simulink library "dpd_lib"  (Simulink 8.7)
settings: Solver=ode45  StartTime=0.0  StopTime=10.0  RelTol=1e-3
PreLoadFcn:
  | LutContent = LUTS.ENTRIES;
InitFcn:
  | LutContent = LUTS.ENTRIES;
undefined symbols (not defined in the file): AdvDSPBChannelOutDisplay, AdvDSPBDMemDisplay, cordic_gain, dpoly, dspba_ChannelInVis, dspba_ChannelOutVis, dspba_internal_get_channel_ports, evalAionMaskParam, latency, LUTS, primtype, UseDontCare, value
libraries: DSPBAPrim x49, dpd_lib x33, DSPBAVectorUtil x2, DSPBABase x1, CORDIC_lib x1
settings Model: Creator=VMAUER  LastModifiedBy=5g

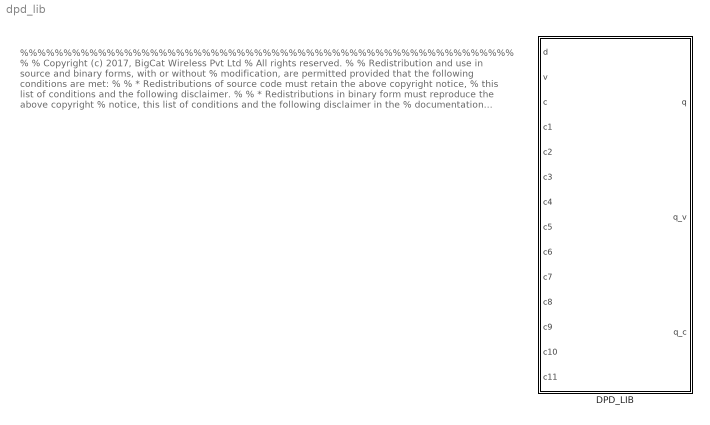
== system dpd_lib ==
  note: %%%%%%%%%%%%%%%%%%%%%%%%%%%%%%%%%%%%%%%%%%%%%%%%%%%%%%%%%
      |  %
      |  % Copyright (c) 2017, BigCat Wireless Pvt Ltd
      |  % All rights reserved.
      |  %
      |  % Redistribution and use in source and binary forms, with or without
      |  % modification, are permitted provided that the following conditions are met:
      |  %
      |  %     * Redistributions of source code must retain the above copyright notice,
      |  %       this list of conditions and the following disclaimer.
      |  %
      |  %     * Redistributions in binary form must reproduce the above copyright
      |  %       notice, this list of conditions and the following disclaimer in the
      |  %       documentation and/or other materials provided with the distribution.
      |  %
      |  %     * Neither the name of the copyright holder nor the names of its contributors
      |  %       may be used to endorse or promote products derived from this software
      |  %       without specific prior written permission.
      |  %
      |  %
      |  %
      |  % THIS SOFTWARE IS PROVIDED BY THE COPYRIGHT HOLDERS AND CONTRIBUTORS "AS IS"
      |  % AND ANY EXPRESS OR IMPLIED WARRANTIES, INCLUDING, BUT NOT LIMITED TO, THE
      |  % IMPLIED WARRANTIES OF MERCHANTABILITY AND FITNESS FOR A PARTICULAR PURPOSE ARE
      |  % DISCLAIMED. IN NO EVENT SHALL THE COPYRIGHT HOLDER OR CONTRIBUTORS BE LIABLE
      |  % FOR ANY DIRECT, INDIRECT, INCIDENTAL, SPECIAL, EXEMPLARY, OR CONSEQUENTIAL
      |  % DAMAGES (INCLUDING, BUT NOT LIMITED TO, PROCUREMENT OF SUBSTITUTE GOODS OR
      |  % SERVICES; LOSS OF USE, DATA, OR PROFITS; OR BUSINESS INTERRUPTION) HOWEVER
      |  % CAUSED AND ON ANY THEORY OF LIABILITY, WHETHER IN CONTRACT, STRICT LIABILITY,
      |  % OR TORT (INCLUDING NEGLIGENCE OR OTHERWISE) ARISING IN ANY WAY OUT OF THE USE
      |  % OF THIS SOFTWARE, EVEN IF ADVISED OF THE POSSIBILITY OF SUCH DAMAGE.
      |  %
      |   %%%%%%%%%%%%%%%%%%%%%%%%%%%%%%%%%%%%%%%%%%%%%%%%%%%%%%%%%%
  DPD_LIB : Subsystem  mask{CoefWidth=16, Coeff_fractionwidth=11, DataWidth=16, fractionwidth=15, Lateny=0, ClockMargin=0, Pipeline_stages=0, LutContent=0}
      mask prompts: CoefWidth "Coefficient Width"; DataWidth "Data Width"; LutContent "initial Lut Content"
      mask Display:
      | disp('DPD');
      | port_label('input',1,'d');
      | port_label('input',2,'v');
      | port_label('input',3,'c');
      | port_label('input',4,'coeffs1');
      | port_label('input',5,'coeffs2');
      | port_label('input',6,'coeffs3');
      | port_label('input',7,'coeffs4');
      | port_label('input',8,'coeffs5');
      | port_label('input',9,'coeffs6');
      | port_label('input',10,'coeffs7');
      | port_label('input',11,'coeffs8');
      | port_label('input',12,'LUTAddress');
      | port_label('input',13,'RegField1');
      | port_label('input',14,'Predistorter_Enable');
      | port_label('output',1,'q');
      | port_label('output',2,'q_v');
      | port_label('output',3,'q_c');

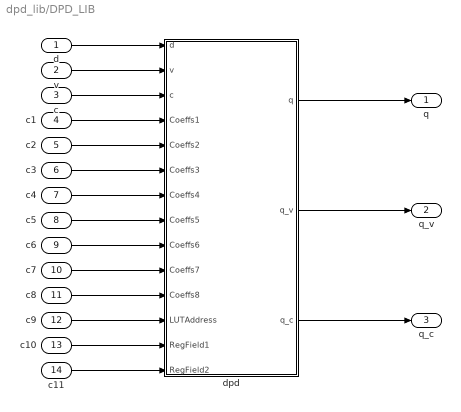
== system dpd_lib/DPD_LIB ==
  d : Inport
  v : Inport  Port=2
  c : Inport  Port=3
  c1 : Inport  Port=4
  c2 : Inport  Port=5
  c3 : Inport  Port=6
  c4 : Inport  Port=7
  c5 : Inport  Port=8
  c6 : Inport  Port=9
  c7 : Inport  Port=10
  c8 : Inport  Port=11
  c9 : Inport  Port=12
  c10 : Inport  Port=13
  c11 : Inport  Port=14
  dpd : Subsystem
  q : Outport
  q_v : Outport  Port=2
  q_c : Outport  Port=3
  wires:
  c/1 -> dpd/3(c)
  d/1 -> dpd/1(d)
  v/1 -> dpd/2(v)
  dpd/1(q) -> q/1
  dpd/2(q_v) -> q_v/1
  dpd/3(q_c) -> q_c/1
  c1/1 -> dpd/4(Coeffs1)
  c2/1 -> dpd/5(Coeffs2)
  c3/1 -> dpd/6(Coeffs3)
  c4/1 -> dpd/7(Coeffs4)
  c5/1 -> dpd/8(Coeffs5)
  c6/1 -> dpd/9(Coeffs6)
  c7/1 -> dpd/10(Coeffs7)
  c10/1 -> dpd/13(RegField1)
  c9/1 -> dpd/12(LUTAddress)
  c8/1 -> dpd/11(Coeffs8)
  c11/1 -> dpd/14(RegField2)

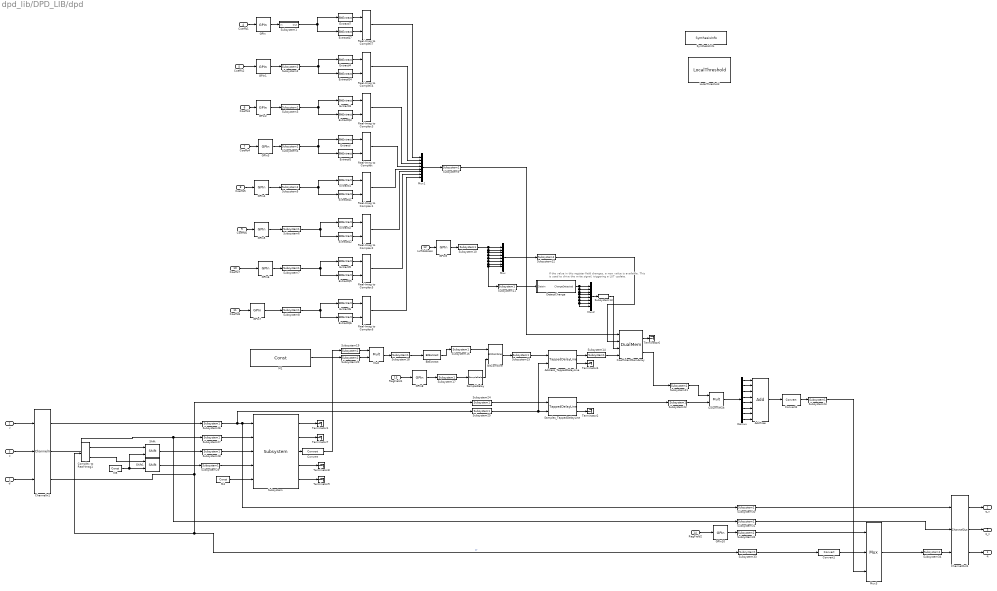
== system dpd_lib/DPD_LIB/dpd ==
  note: If the value in this register field changes, a new value is available.
      | This is used to drive the write signal, triggering a LUT update.
  d : Inport
  v : Inport  Port=2
  c : Inport  Port=3
  Coeffs1 : Inport  Port=4
  Coeffs2 : Inport  Port=5
  Coeffs3 : Inport  Port=6
  Coeffs4 : Inport  Port=7
  Coeffs5 : Inport  Port=8
  Coeffs6 : Inport  Port=9
  Coeffs7 : Inport  Port=10
  Coeffs8 : Inport  Port=11
  LUTAddress : Inport  Port=12
  RegField1 : Inport  Port=13
  RegField2 : Inport  Port=14
  AddTree : DSPBAPrim/Add  primtype=add  nInputs=evalAionMaskParam(gcb,'value',1)  nOutputs=1  omode=Inherit via internal rule with word growth  otype=sfix(16)  scale=2^-15  rndmethod=Unbiased  factor=1  satmethod=Symmetric  shift_vec=[0 1 2 -1]  value=8  inPortNames=[' '; ' ';]  outPortNames=[' ']  dspbaimage=dspba_prim.jpg  text=fprintf('+');  style=Optimised  visibilities=1032+2^17+2^18+2^19  genFPC=off  floatRounding=correct  advOptions=[]  version=20130821
  Address_TappedDelayLine : DSPBAVectorUtil/TappedDelayLine  numTaps=size(LutContent, 2)  zeroOrOne=0  reverse=off
  BitCombine : DSPBAPrim/BitCombine  primtype=bitcombine  nInputs=2  nOutputs=1  omode=Inherit via internal rule  otype=sfix(16)  scale=2^-15  rndmethod=Unbiased  factor=1  satmethod=Symmetric  shift_vec=[0 1 2 -1]  value=0  inPortNames=['l'; 'h';]  outPortNames=[' ']  dspbaimage=dspba_prim.jpg  text=fprintf('[h,l]');  style=Optimised  visibilities=8+2  version=20090407
  BitExtract : DSPBAPrim/BitExtract  primtype=bitextract  nInputs=1  nOutputs=1  omode=Specify via dialog  otype=ufix(8)  scale=1  rndmethod=Unbiased  factor=1  satmethod=Symmetric  shift_vec=[0 1 2 -1]  value=log2(size(LutContent,1))  inPortNames=[' '; ' ';]  outPortNames=[' ']  dspbaimage=dspba_prim.jpg  text=fprintf('..%d', value);  style=Optimised  visibilities=8 + 1024  version=20090407
  ChannelIn1 : DSPBAPrim/ChannelIn  primtype=channelin  nInputs=dspba_internal_get_channel_ports(gcb)  nOutputs=dspba_internal_get_channel_ports(gcb)  omode=Inherit via internal rule  otype=sfix(16)  scale=2^-15  rndmethod=Unbiased  factor=1  satmethod=Symmetric  shift_vec=[0 1 2 -1]  value=1  inPortNames=['v'; 'c'; '0'; '1'; '2'; '3'; '4'; '5'; '6'; '7'; '8'; '9'; 'A'; 'B'; 'D'; 'E'; 'F'; 'G'; 'H'; 'I'; 'J'; 'K'; 'L'; 'M'; 'N'; 'O'; 'P'; 'Q'; 'R'; 'S'; 'T'; 'U'; 'W'; 'X'; 'Y'; 'Z']  outPortNames=['v'; 'c'; '0'; '1'; '2'; '3'; '4'; '5'; '6'; '7'; '8'; '9'; 'A'; 'B'; 'D'; 'E'; 'F'; 'G'; 'H'; 'I'; 'J'; 'K'; 'L'; 'M'; 'N'; 'O'; 'P'; 'Q'; 'R'; 'S'; 'T'; 'U'; 'W'; 'X'; 'Y'; 'Z']  dspbaimage=dspba_prim.jpg  text=fprintf('In');  style=Optimised  dataSignals=1  foldingEnabled=off  channels=1  sampleRate=200  packetBeginPresent=off  packetBeginEnabled=off  visibilities=dspba_ChannelInVis(gcb)  latencyCorrection=0  version=20141013
  ChannelOut1 : DSPBAPrim/ChannelOut  primtype=channelout  nInputs=dspba_internal_get_channel_ports(gcb)  nOutputs=dspba_internal_get_channel_ports(gcb)  omode=Inherit via internal rule  otype=sfix(16)  scale=2^-15  rndmethod=Unbiased  factor=1  satmethod=Symmetric  shift_vec=[0 1 2 -1]  value=1  inPortNames=['v'; 'c'; '0'; '1'; '2'; '3'; '4'; '5'; '6'; '7'; '8'; '9'; 'A'; 'B'; 'D'; 'E'; 'F'; 'G'; 'H'; 'I'; 'J'; 'K'; 'L'; 'M'; 'N'; 'O'; 'P'; 'Q'; 'R'; 'S'; 'T'; 'U'; 'W'; 'X'; 'Y'; 'Z']  outPortNames=['v'; 'c'; '0'; '1'; '2'; '3'; '4'; '5'; '6'; '7'; '8'; '9'; 'A'; 'B'; 'D'; 'E'; 'F'; 'G'; 'H'; 'I'; 'J'; 'K'; 'L'; 'M'; 'N'; 'O'; 'P'; 'Q'; 'R'; 'S'; 'T'; 'U'; 'W'; 'X'; 'Y'; 'Z']  dspbaimage=dspba_prim.jpg  text=fprintf('Out%s', AdvDSPBChannelOutDisplay(latency));  style=Optimised  dataSignals=1  foldingEnabled=off  channels=1  sampleRate=200  packetBeginPresent=off  packetBeginEnabled=off  visibilities=dspba_ChannelOutVis(gcb)  latency=101  latencyCorrection=0  version=20141013
  CoefficientMemArray : DSPBAPrim/DualMem  primtype=dualmem  nInputs=4  nOutputs=2  omode=Specify via dialog  otype=sfix(CoefWidth)  scale=2^-Coeff_fractionwidth  rndmethod=Unbiased  factor=1  satmethod=Symmetric  shift_vec=[0 1 2 -1]  value=[LUTS.ENTRIES' LUTS.ENTRIES']'  inPortNames=['d1'; 'a1'; 'w1'; 'a2']  outPortNames=['q1'; 'q2']  dspbaimage=dspba_prim.jpg  text=fprintf('dmem%s',AdvDSPBDMemDisplay(UseDontCare));  style=Optimised  visibilities=8 + 1024 + 2^17  UseDontCare=on  TwinWritePorts=off  version=20141001
  ColumnMult : DSPBAPrim/Mult  primtype=mult  nInputs=2  nOutputs=1  omode=Inherit via internal rule  otype=sfix(16)  scale=2^-11  rndmethod=Unbiased  factor=1  satmethod=Symmetric  shift_vec=[0 1 2 -1]  value=0  inPortNames=[' '; ' ';]  outPortNames=[' ']  dspbaimage=dspba_prim.jpg  text=fprintf('X');  style=Optimised  visibilities=8+2^18+2^19  floatPrecision=float32_m23  floatRounding=correct  advOptions=[]  version=20130115
  Complex to Real-Imag1 : ComplexToRealImag
  Convert : DSPBAPrim/Convert  primtype=convert  nInputs=1  nOutputs=1  omode=Specify via dialog  otype=ufix(10)  scale=2^-8  rndmethod=Truncate  factor=1  satmethod=None  shift_vec=[0 1 2 -1]  value=round([0:255]/17)  inPortNames=[' '; ' ';]  outPortNames=[' '; 'c']  dspbaimage=dspba_prim.jpg  text=fprintf('convert');  style=Optimised  visibilities=8+64+256+2^17  clipdetect=off  floatPrecision=float32_m23  advOptions=[]  version=20130211
  Convert1 : DSPBAPrim/Convert  primtype=convert  nInputs=1  nOutputs=1  omode=Specify via dialog  otype=sfix(16)  scale=2^-15  rndmethod=Unbiased  factor=1  satmethod=None  shift_vec=[0 1 2 -1]  value=round([0:255]/17)  inPortNames=[' '; ' ';]  outPortNames=[' '; 'c']  dspbaimage=dspba_prim.jpg  text=fprintf('convert');  style=Optimised  visibilities=8+64+256+2^17  clipdetect=off  floatPrecision=float32_m23  advOptions=[]  version=20130211
  Convert2 : DSPBAPrim/Convert  primtype=convert  nInputs=1  nOutputs=1  omode=Specify via dialog  otype=sfix(DataWidth)  scale=2^-fractionwidth  rndmethod=Unbiased  factor=1  satmethod=None  shift_vec=[0 1 2 -1]  value=round([0:255]/17)  inPortNames=[' '; ' ';]  outPortNames=[' '; 'c']  dspbaimage=dspba_prim.jpg  text=fprintf('convert');  style=Optimised  visibilities=8+64+256  clipdetect=off  floatPrecision=float32_m23  advOptions=[]  version=20130211
  Demux : Demux  Outputs=8
  DetectChange : Subsystem
  ExtractI{,1..7} (8 alike) : DSPBAPrim/BitExtract  primtype=bitextract  nInputs=1  nOutputs=1  omode=Specify via dialog  otype=sfix(CoefWidth)  scale=2^-Coeff_fractionwidth  rndmethod=Unbiased  factor=1  satmethod=Symmetric  shift_vec=[0 1 2 -1]  value=CoefWidth  inPortNames=[' '; ' ';]  outPortNames=[' ']  dspbaimage=dspba_prim.jpg  text=fprintf('..%d', value);  style=Optimised  visibilities=8 + 1024  version=20090407
  ExtractQ{,1..3,5..6} (6 alike) : DSPBAPrim/BitExtract  primtype=bitextract  nInputs=1  nOutputs=1  omode=Specify via dialog  otype=sfix(CoefWidth)  scale=2^-Coeff_fractionwidth  rndmethod=Unbiased  factor=1  satmethod=Symmetric  shift_vec=[0 1 2 -1]  value=0  inPortNames=[' '; ' ';]  outPortNames=[' ']  dspbaimage=dspba_prim.jpg  text=fprintf('..%d', value);  style=Optimised  visibilities=8 + 1024  version=20090407
  ExtractQ4 : DSPBAPrim/BitExtract  primtype=bitextract  nInputs=1  nOutputs=1  omode=Specify via dialog  otype=sfix(DataWidth)  scale=2^-Coeff_fractionwidth  rndmethod=Unbiased  factor=1  satmethod=Symmetric  shift_vec=[0 1 2 -1]  value=0  inPortNames=[' '; ' ';]  outPortNames=[' ']  dspbaimage=dspba_prim.jpg  text=fprintf('..%d', value);  style=Optimised  visibilities=8 + 1024  version=20090407
  ExtractQ7 : DSPBAPrim/BitExtract  primtype=bitextract  nInputs=1  nOutputs=1  omode=Specify via dialog  otype=sfix(DataWidth)  scale=2^-Coeff_fractionwidth  rndmethod=Unbiased  factor=1  satmethod=Symmetric  shift_vec=[0 1 2 -1]  value=0  inPortNames=[' '; ' ';]  outPortNames=[' ']  dspbaimage=dspba_prim.jpg  text=fprintf('..%d', value);  style=Optimised  visibilities=8 + 1024  version=20090407
  GPIn{,1..10} (11 alike) : DSPBAPrim/GPIn  primtype=gpin  nInputs=evalAionMaskParam(gcb,'value',1)  nOutputs=evalAionMaskParam(gcb,'value',1)  omode=Inherit via internal rule  otype=sfix(16)  scale=2^-15  rndmethod=Unbiased  factor=1  satmethod=Symmetric  shift_vec=[0 1 2 -1]  value=1  inPortNames=[' ' ' ' ' ' ' ' ' ' ' ' ' ' ' ' ' ' ' ' ' ' ' ' ' ' ' ' ' ' ' ' ' ' ' ' ' ' ' ' ' ' ' ' ' ' ' ' ' ' ' ' ' ' ' ' ' ' ' ' ' ' ' ' ' ' ' ' ' ']'  outPortNames=[' ' ' ' ' ' ' ' ' ' ' ' ' ' ' ' ' ' ' ' ' ' ' ' ' ' ' ' ' ' ' ' ' ' ' ' ' ' ' ' ' ' ' ' ' ' ' ' ' ' ' ' ' ' ' ' ' ' ' ' ' ' ' ' ' ' ' ' ' ']'  dspbaimage=dspba_prim.jpg  text=fprintf('GPIn');  style=Optimised  visibilities=1024  latencyCorrection=0  version=20090407
  LocalThreshold : DSPBABase/LocalThreshold  margin=ClockMargin  delayRegOrRAMThresholdBits=-1  MediumDualMemThresholdBits=-1  LargeDualMemThresholdBits=-1  hardMultiplierThresholdLuts=-1  complexMultKaratsuba=off  version=0
  M1 : DSPBAPrim/Const  primtype=const  nInputs=0  nOutputs=1  omode=Specify via dialog  otype=uint(8)  scale=1  rndmethod=Unbiased  factor=1  satmethod=Symmetric  shift_vec=[0 1 2 -1]  value=size(LutContent, 1) * (1/cordic_gain)  inPortNames=['+'; '+';]  outPortNames=[' ']  dspbaimage=dspba_prim.jpg  text=fprintf('%s', num2str(value));  style=Optimised  visibilities=8 + 1024  floatPrecision=float32_m23  version=20120820
  M4 : DSPBAPrim/Const  primtype=const  nInputs=0  nOutputs=1  omode=Specify via dialog  otype=sfix(16)  scale=2^-15  rndmethod=Unbiased  factor=1  satmethod=Symmetric  shift_vec=[0 1 2 -1]  value=0  inPortNames=['+'; '+';]  outPortNames=[' ']  dspbaimage=dspba_prim.jpg  text=fprintf('%s', num2str(value));  style=Optimised  visibilities=8 + 1024  floatPrecision=float32_m23  version=20120820
  M5 : DSPBAPrim/Const  primtype=const  nInputs=0  nOutputs=1  omode=Specify via dialog  otype=uint(4)  scale=2^0  rndmethod=Unbiased  factor=1  satmethod=Symmetric  shift_vec=[0 1 2 -1]  value=2  inPortNames=['+'; '+';]  outPortNames=[' ']  dspbaimage=dspba_prim.jpg  text=fprintf('%s', num2str(value));  style=Optimised  visibilities=8 + 1024  floatPrecision=float32_m23  version=20120820
  Mult : DSPBAPrim/Mult  primtype=mult  nInputs=2  nOutputs=1  omode=Inherit via internal rule  otype=double  scale=1  rndmethod=Unbiased  factor=1  satmethod=Symmetric  shift_vec=[0 1 2 -1]  value=0  inPortNames=[' '; ' ';]  outPortNames=[' ']  dspbaimage=dspba_prim.jpg  text=fprintf('X');  style=Optimised  visibilities=8  floatPrecision=float32_m23  floatRounding=correct  advOptions=[]  version=20130115
  Mux : Mux  Inputs=8
  Mux1 : Mux  Inputs=8
  Mux2 : Mux  Inputs=8
  Mux3 : DSPBAPrim/Mux  primtype=mux  nInputs=evalAionMaskParam(gcb,'value',1)+1  nOutputs=1  omode=Inherit via internal rule  otype=sfix(16)  scale=2^-15  rndmethod=Unbiased  factor=1  satmethod=Symmetric  shift_vec=[0 1 2 -1]  value=2  inPortNames=['s'; 'd0'; 'd1'; 'd2'; 'd3'; 'd4'; 'd5'; 'd6'; 'd7'; 'd8'; 'd9';]  outPortNames=[' ']  dspbaimage=dspba_prim.jpg  text=fprintf('%s', primtype);  style=Optimised  visibilities=1032  version=20131025
  Real-Imag to Complex{,1..7} (8 alike) : RealImagToComplex
  SampleDelay : DSPBAPrim/SampleDelay  primtype=sampdelay  nInputs=1  nOutputs=1  omode=Inherit via internal rule  otype=sfix(16)  scale=2^-15  rndmethod=Unbiased  factor=1  satmethod=Symmetric  shift_vec=[0 1 2 -1]  value=1  inPortNames=[' '; ' ';]  outPortNames=[' ']  dspbaimage=dspba_prim.jpg  text=dpoly(1, eye(1,value+1), 'z')  style=Optimised  visibilities=8 + 1024 + 2^17 + 2^18  flexible=off  slackgroup=0  augmented=0  version=20090407  advOptions=[]
  Samples_TappedDelayLine : DSPBAVectorUtil/TappedDelayLine  numTaps=size(LutContent, 2)  zeroOrOne=0  reverse=off
  Shift : DSPBAPrim/Shift  primtype=shift  nInputs=2  nOutputs=1  omode=Specify via dialog  otype=sfix(16)  scale=2^-15  rndmethod=Unbiased  factor=1  satmethod=Symmetric  shift_vec=[0 1 2 -1]  value=0  inPortNames=['a'; 'b';]  outPortNames=[' ']  dspbaimage=dspba_prim.jpg  text=fprintf('a >> b');  style=Optimised  visibilities=8  version=20090407
  Shift1 : DSPBAPrim/Shift  primtype=shift  nInputs=2  nOutputs=1  omode=Specify via dialog  otype=sfix(16)  scale=2^-15  rndmethod=Unbiased  factor=1  satmethod=Symmetric  shift_vec=[0 1 2 -1]  value=0  inPortNames=['a'; 'b';]  outPortNames=[' ']  dspbaimage=dspba_prim.jpg  text=fprintf('a >> b');  style=Optimised  visibilities=8  version=20090407
  Subsystem : CORDIC_lib/Subsystem  stages=stages  angle_bits=xy_angle_bits  angle_frac_bits=xy_angle_fract_bits  xy_bits=xy_bits  xy_frac_bits=xy_fract_bits
  Subsystem1 : Subsystem
  Subsystem{2..34} (33 alike) : dpd_lib/DPD_LIB/dpd/Subsystem1
  SynthesisInfo : DSPBAPrim/SynthesisInfo  primtype=synthinfo  nInputs=0  nOutputs=0  omode=Inherit via internal rule  otype=sfix(16)  scale=2^-15  rndmethod=Truncate  factor=1  satmethod=Symmetric  shift_vec=[0 1 2 -1]  value=99  inPortNames=[' '; ' ';]  outPortNames=[' ']  dspbaimage=dspba_prim_ctrl.jpg  text=fprintf('Style=%s', style);  style=Scheduled  visibilities=2^15+2^17+2^18+2^19  constraintInUse=on  constraintRelation=>  constraintLimit=Lateny  bitAccurate=off  version=20150220
  Terminator{1..2,4,6..9} (7 alike) : Terminator
  q : Outport
  q_v : Outport  Port=2
  q_c : Outport  Port=3
  wires:
  ExtractI2/1 -> Real-Imag to Complex2/1
  ExtractQ2/1 -> Real-Imag to Complex2/2
  ExtractI3/1 -> Real-Imag to Complex3/1
  ExtractQ3/1 -> Real-Imag to Complex3/2
  ExtractI4/1 -> Real-Imag to Complex4/1
  ExtractQ4/1 -> Real-Imag to Complex4/2
  Subsystem/2 -> Terminator7/1
  ExtractI5/1 -> Real-Imag to Complex5/1
  ExtractQ5/1 -> Real-Imag to Complex5/2
  ExtractI6/1 -> Real-Imag to Complex6/1
  ExtractQ6/1 -> Real-Imag to Complex6/2
  ExtractI7/1 -> Real-Imag to Complex7/1
  ExtractQ7/1 -> Real-Imag to Complex7/2
  Real-Imag to Complex/1 -> Mux1/4
  Real-Imag to Complex1/1 -> Mux1/5
  DetectChange/1(ChangeDetected) -> Mux2/2, Mux2/3, Mux2/4, Mux2/5, Mux2/6, Mux2/7, Mux2/8, Mux2/1
  Real-Imag to Complex2/1 -> Mux1/6
  Real-Imag to Complex5/1 -> Mux1/7
  Real-Imag to Complex6/1 -> Mux1/8
  Real-Imag to Complex3/1 -> Mux1/3
  Real-Imag to Complex4/1 -> Mux1/2
  Real-Imag to Complex7/1 -> Mux1/1
  Mux1/1 -> Subsystem9/1
  Mux2/1 -> Subsystem13/1
  ColumnMult/1 -> Demux/1
  Demux/1 -> AddTree/1
  Demux/2 -> AddTree/2
  Demux/3 -> AddTree/3
  Demux/4 -> AddTree/4
  Demux/5 -> AddTree/5
  Convert1/1 -> Mux3/2
  Subsystem32/1 -> Mux3/1
  d/1 -> ChannelIn1/3
  ChannelIn1/2 -> Subsystem31/1, Subsystem27/1
  Convert2/1 -> Subsystem23/1
  ChannelIn1/1 -> Subsystem26/1
  v/1 -> ChannelIn1/1
  Samples_TappedDelayLine/2 -> Terminator2/1
  ChannelOut1/3 -> q/1
  Demux/6 -> AddTree/6
  Demux/7 -> AddTree/7
  Demux/8 -> AddTree/8
  M4/1 -> Subsystem/5
  Subsystem/1 -> Terminator1/1
  Subsystem/4 -> Terminator8/1
  Subsystem/5 -> Terminator9/1
  Mult/1 -> Subsystem18/1
  Subsystem/3 -> Convert/1
  Convert/1 -> Subsystem19/1
  SampleDelay/1 -> BitCombine/2
  Subsystem10/1 -> Mux/4, Mux/5, Mux/6, Mux/7, Subsystem11/1, Mux/8, Mux/3, Mux/2, Mux/1
  Shift/1 -> Subsystem28/1
  Shift1/1 -> Subsystem29/1
  M5/1 -> Shift/2, Shift1/2
  Mux3/1 -> Subsystem34/1
  CoefficientMemArray/1 -> Terminator6/1
  Complex to Real-Imag1/1 -> Shift/1
  Complex to Real-Imag1/2 -> Shift1/1
  Address_TappedDelayLine/2 -> Terminator4/1
  CoefficientMemArray/2 -> Subsystem21/1
  AddTree/1 -> Convert2/1
  Samples_TappedDelayLine/1 -> Subsystem22/1
  BitCombine/1 -> Subsystem15/1
  Address_TappedDelayLine/1 -> Subsystem14/1
  ExtractI/1 -> Real-Imag to Complex/1
  ExtractQ/1 -> Real-Imag to Complex/2
  M1/1 -> Subsystem20/1
  BitExtract/1 -> Subsystem16/1
  Mux/1 -> Subsystem12/1
  ExtractI1/1 -> Real-Imag to Complex1/1
  ExtractQ1/1 -> Real-Imag to Complex1/2
  c/1 -> ChannelIn1/2
  ChannelIn1/3 -> Subsystem24/1, Subsystem33/1, Complex to Real-Imag1/1  "xr"
  ChannelOut1/1 -> q_v/1
  ChannelOut1/2 -> q_c/1
  Subsystem23/1 -> Mux3/3
  Subsystem30/1 -> ChannelOut1/1
  Subsystem31/1 -> ChannelOut1/2
  Subsystem33/1 -> Convert1/1
  Subsystem34/1 -> ChannelOut1/3
  Subsystem21/1 -> ColumnMult/1
  Subsystem22/1 -> ColumnMult/2
  Subsystem14/1 -> CoefficientMemArray/4
  Subsystem15/1 -> Address_TappedDelayLine/1
  Subsystem16/1 -> BitCombine/1
  Subsystem17/1 -> SampleDelay/1
  Subsystem24/1 -> Samples_TappedDelayLine/1
  Subsystem25/1 -> Address_TappedDelayLine/2, Samples_TappedDelayLine/2
  Subsystem18/1 -> BitExtract/1
  Subsystem19/1 -> Mult/1
  Subsystem20/1 -> Mult/2
  Subsystem27/1 -> Subsystem/2
  Subsystem28/1 -> Subsystem/3
  Subsystem29/1 -> Subsystem/4
  Subsystem26/1 -> Subsystem25/1, Subsystem30/1, Subsystem/1
  Subsystem9/1 -> CoefficientMemArray/1
  Subsystem12/1 -> CoefficientMemArray/2
  Subsystem13/1 -> CoefficientMemArray/3
  Subsystem11/1 -> DetectChange/1(DataIn)
  Coeffs1/1 -> GPIn/1
  Subsystem2/1 -> ExtractI4/1, ExtractQ4/1
  Coeffs2/1 -> GPIn1/1
  Subsystem3/1 -> ExtractI3/1, ExtractQ3/1
  Coeffs3/1 -> GPIn2/1
  Subsystem4/1 -> ExtractI/1, ExtractQ/1
  Coeffs4/1 -> GPIn3/1
  Subsystem5/1 -> ExtractQ1/1, ExtractI1/1
  Coeffs5/1 -> GPIn4/1
  Subsystem6/1 -> ExtractQ2/1, ExtractI2/1
  Coeffs6/1 -> GPIn5/1
  Subsystem7/1 -> ExtractQ5/1, ExtractI5/1
  Coeffs7/1 -> GPIn6/1
  Subsystem8/1 -> ExtractQ6/1, ExtractI6/1
  Coeffs8/1 -> GPIn7/1
  LUTAddress/1 -> GPIn9/1
  RegField1/1 -> GPIn8/1
  GPIn1/1 -> Subsystem2/1
  GPIn2/1 -> Subsystem3/1
  GPIn3/1 -> Subsystem4/1
  GPIn4/1 -> Subsystem5/1
  GPIn5/1 -> Subsystem6/1
  GPIn6/1 -> Subsystem7/1
  GPIn7/1 -> Subsystem8/1
  GPIn8/1 -> Subsystem17/1
  GPIn9/1 -> Subsystem10/1
  RegField2/1 -> GPIn10/1
  GPIn10/1 -> Subsystem32/1
  Subsystem1/1(Out) -> ExtractQ7/1, ExtractI7/1
  GPIn/1 -> Subsystem1/1(In)

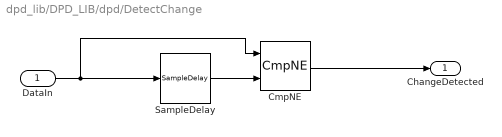
== system dpd_lib/DPD_LIB/dpd/DetectChange ==
  DataIn : Inport
  CmpNE : DSPBAPrim/CmpNE  primtype=cmpne  nInputs=2  nOutputs=1  omode=boolean  otype=sfix(16)  scale=2^-15  rndmethod=Unbiased  factor=1  satmethod=Symmetric  shift_vec=[0 1 2 -1]  value=0  inPortNames=[' '; ' ';]  outPortNames=[' ']  dspbaimage=dspba_prim.jpg  text=fprintf('~=');  style=Optimised  visibilities=0  advOptions=[]  version=20130117
  SampleDelay : DSPBAPrim/SampleDelay  primtype=sampdelay  nInputs=1  nOutputs=1  omode=Inherit via internal rule  otype=sfix(16)  scale=2^-15  rndmethod=Unbiased  factor=1  satmethod=Symmetric  shift_vec=[0 1 2 -1]  value=1  inPortNames=[' '; ' ';]  outPortNames=[' ']  dspbaimage=dspba_prim.jpg  text=dpoly(1, eye(1,value+1), 'z')  style=Optimised  visibilities=8 + 1024 + 2^17 + 2^18  flexible=off  slackgroup=0  augmented=0  version=20090407  advOptions=[]
  ChangeDetected : Outport
  wires:
  CmpNE/1 -> ChangeDetected/1
  DataIn/1 -> CmpNE/1, SampleDelay/1
  SampleDelay/1 -> CmpNE/2

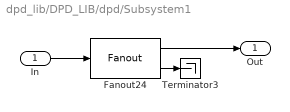
== system dpd_lib/DPD_LIB/dpd/Subsystem1 ==
  In : Inport
  Fanout24 : DSPBAPrim/Fanout  primtype=fanout  nInputs=1  nOutputs=evalAionMaskParam(gcb,'value',1)  omode=Inherit via internal rule  otype=sfix(16)  scale=2^-15  rndmethod=Unbiased  factor=1  satmethod=Symmetric  shift_vec=[0 1 2 -1]  value=2  inPortNames=[' '; ' ';]  outPortNames=[' ']  dspbaimage=dspba_prim.jpg  text=fprintf('fanout')  style=Optimised  visibilities=2^10+2^18  version=20150501  uninit=off
  Terminator3 : Terminator
  Out : Outport
  wires:
  Fanout24/2 -> Terminator3/1
  Fanout24/1 -> Out/1
  In/1 -> Fanout24/1
